simulink model "DIL_brute_force"  (R2023b)
settings: Solver=VariableStepAuto  StartTime=0.0  StopTime=10.0  RelTol=1e-3
values from neighbouring files (symbols this model uses):
  dt = 0.01    [setup.m]
  optsODE = odeset('Mass',M, 'AbsTol', 1e-3, 'RelTol', 1e-3)    [DIL_matlab.m]    (also in setup.m = odeset('Mass',M,'RelTol',1e-2, 'AbsTol', 1e-2))
  s0 = load("s0.mat").s1(1:22)    [DIL_matlab.m]    (also in setup.m = [0; 0; 0; 0; 0; varCAR.z0(1) + varCAR.L0(1) - varCAR.LN - 0.)
  varCAR = class2struct(vehicle_parameters)    [DIL_matlab.m]    (also in setup.m = class2struct(varCAR))
settings Model: Creator=Inver  LastModifiedBy=Inver

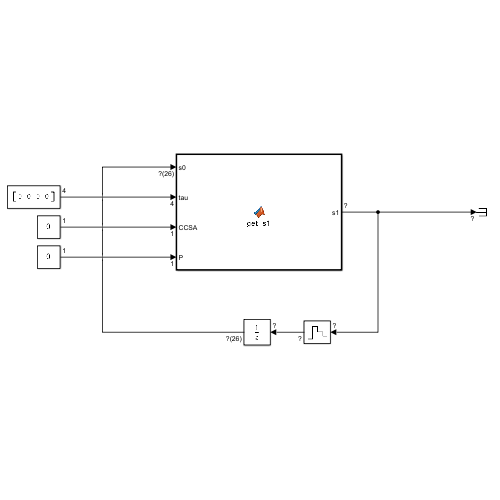
[thumbnail: Simulink's stored preview of the top-level diagram]
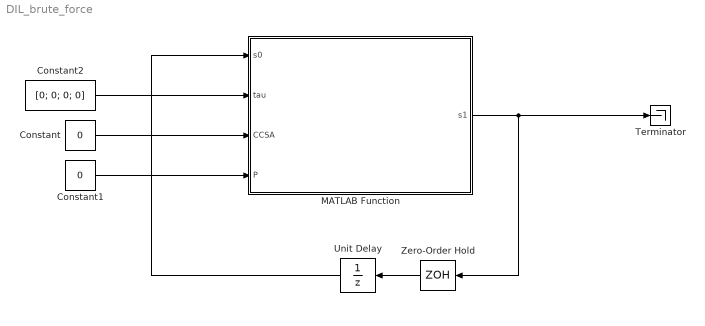
== system DIL_brute_force ==
  Constant : Constant  Value=0
  Constant1 : Constant  Value=0
  Constant2 : Constant  Value=[0; 0; 0; 0]
  MATLAB Function : MATLAB Function  TreatAsAtomicUnit=on  SystemSampleTime=dt
  Terminator : Terminator
  Unit Delay : UnitDelay  InitialCondition=s0  SampleTime=dt  HasFrameUpgradeWarning=on
  Zero-Order Hold : ZeroOrderHold  SampleTime=dt
  wires:
  MATLAB Function/1(s1) -> Zero-Order Hold/1, Terminator/1
  Zero-Order Hold/1 -> Unit Delay/1
  Unit Delay/1 -> MATLAB Function/1(s0)
  Constant/1 -> MATLAB Function/3(CCSA)
  Constant1/1 -> MATLAB Function/4(P)
  Constant2/1 -> MATLAB Function/2(tau)

== matlab function DIL_brute_force/MATLAB Function ==
  data: s0 input; s1 output; tau input; CCSA input; P input; varCAR parameter; dt parameter; optsODE parameter
function s1 = get_s1(s0, tau, CCSA, P, varCAR, dt, optsODE)
    [t,s] = ode15s(@vehicle_ds, [0 dt], s0, optsODE, tau, CCSA, P, varCAR);
    s1 = s(end,:);
end
